simulink model "GCI_Ctrl_PLL_C2000"  (R2024a)
settings: Solver=FixedStepDiscrete  StartTime=0.0  StopTime=8  FixedStep=Sim.ContSampleTime  RelTol=1e-3  EnableMultiTasking=on
values from neighbouring files (symbols this model uses):
  ADPTV = 1.3912    [ModelDD.sldd]
  Ctrl = 0    [ModelDD.sldd]
  EnableMonitors = 0    [ModelDD.sldd]
  FrcPwr = 1    [ModelDD.sldd]
  IdSp = 0.0    [ModelDD.sldd]
  IqSp = 0.0    [ModelDD.sldd]
  ModReq = 1    [ModelDD.sldd]
  PorISel = 0    [ModelDD.sldd]
  PSp = 0.0    [ModelDD.sldd]
  QSp = 0.0    [ModelDD.sldd]
  Sim : value not decoded    [ModelDD.sldd]
  Test = 0    [ModelDD.sldd]
  Var = 650.0    [ModelDD.sldd]
undefined symbols (not defined in the file or in its folder): DiscIntNeverNeededParam, Down, GPTRIP1SEL, GPTRIP2SEL, magnitude, P, TZ1, TZ2, Up
libraries: simulink x38, c2837xDlib x22, c2802xlib x15, slpidlib x9, spsMeanLib x9, spsCurrentMeasurementLib x7, spsThreePhaseVIMeasurementLib x5, spsVoltageMeasurementLib x5, spsTHDLib x4, spsSeriesRLCBranchLib x4, svdutilitieslib x3, c280xlib x3
(part 10 of 11)

== system GCI_Ctrl_PLL_C2000/C2000_SW/CtrlLoop/CurrentController/CurrentControllerAdptv/Subsystem/dd_dqz1/LPF1 ==
  u : Inport
  Alpha : Gain  Gain=(2-w*Ts)/(2+w*Ts)
  Beta : Gain  Gain=(w*Ts)/(2+w*Ts)
  Delay1 : Delay  DelayLength=1  InitialCondition=y_0
  Delay2 : Delay  DelayLength=1
  Sum1 : Sum  Inputs=++|
  Sum2 : Sum  Inputs=|++
  y : Outport  VectorParamsAs1DForOutWhenUnconnected=off
  wires:
  u/1 -> Sum1/1, Delay2/1
  Delay1/1 -> Alpha/1  "y(n-1)"
  Alpha/1 -> Sum2/2
  Delay2/1 -> Sum1/2
  Sum1/1 -> Beta/1
  Beta/1 -> Sum2/1
  Sum2/1 -> Delay1/1, y/1

== system GCI_Ctrl_PLL_C2000/C2000_SW/CtrlLoop/CurrentController/CurrentControllerAdptv/Subsystem/dd_dqz1/Subsystem ==
  abc : Inport  PortDimensions=3
  Gain1 : Gain  Gain=single(2/3)  ParamDataTypeStr=single  SaturateOnIntegerOverflow=on  OutDataTypeStr=Inherit: Same as input
  Gain3 : Gain  Gain="single([ 1   -1/2   -1/2; 0   sqrt(3)/2   -sqrt(3)/2; 1/2  1/2  1/2 ] )"  Multiplication=Matrix(K*u) (u vector)  ParamDataTypeStr=single  SaturateOnIntegerOverflow=on  OutDataTypeStr=Inherit: Same as input
  al_be_0 : Outport  VectorParamsAs1DForOutWhenUnconnected=off
  wires:
  Gain1/1 -> al_be_0/1  "AlphaBetaZero"
  Gain3/1 -> Gain1/1
  abc/1 -> Gain3/1

== system GCI_Ctrl_PLL_C2000/C2000_SW/CtrlLoop/CurrentController/CurrentControllerAdptv/Subsystem/dd_dqz1/Subsystem1 ==
  note: [  al
      |     be  ]
  note: q = -al*sin(wt) + be*cos(wt)
  note: [  cos(wt)   sin(wt)
      |    -sin(wt)    cos(wt)   ]
  note: d = al*cos(wt) + be*sin(wt)
  note: [ d
      |    q ]
  note: *
  note: =
  alpha_beta : Inport
  wtNow : Inport  Port=2  PortDimensions=1
  Fcn : Fcn  Expr=u[1]*cos(u[3]) + u[2]*sin(u[3])
  Fcn1 : Fcn  Expr=-u[1]*sin(u[3]) + u[2]*cos(u[3])
  Mux : Mux  Inputs=3
  Mux1 : Mux  Inputs=[2 1]
  Mux2 : Mux  Inputs=[2 1]
  Selector : Selector  InputPortWidth=3  IndexOptions=Index vector (dialog)  Indices=[1 2]  OutputSizes=1
  Selector1 : Selector  InputPortWidth=3  IndexOptions=Index vector (dialog)  Indices=[3]  OutputSizes=1
  dq : Outport  InitialOutput=[0,0]  VectorParamsAs1DForOutWhenUnconnected=off
  wires:
  Selector1/1 -> Mux/3
  Selector/1 -> Mux1/1, Mux2/1
  Mux2/1 -> Fcn1/1
  Mux/1 -> dq/1
  wtNow/1 -> Mux1/2, Mux2/2
  Fcn/1 -> Mux/1
  Fcn1/1 -> Mux/2
  Mux1/1 -> Fcn/1
  alpha_beta/1 -> Selector1/1, Selector/1

== system GCI_Ctrl_PLL_C2000/C2000_SW/CtrlLoop/CurrentController/CurrentControllerAdptv/Subsystem/dd_dqz1/Subsystem2 ==
  note: =
  note: *
  note: [ d
      |    q ]
  note: d = al*cos(wt) + be*sin(wt)
  note: [  cos(wt)   sin(wt)
      |    -sin(wt)    cos(wt)   ]
  note: q = -al*sin(wt) + be*cos(wt)
  note: [  al
      |     be  ]
  alpha_beta : Inport
  wtNow : Inport  Port=2  PortDimensions=1
  Fcn : Fcn  Expr=u[1]*cos(u[3]) + u[2]*sin(u[3])
  Fcn1 : Fcn  Expr=-u[1]*sin(u[3]) + u[2]*cos(u[3])
  Mux : Mux  Inputs=3
  Mux1 : Mux  Inputs=[2 1]
  Mux2 : Mux  Inputs=[2 1]
  Selector : Selector  InputPortWidth=3  IndexOptions=Index vector (dialog)  Indices=[1 2]  OutputSizes=1
  Selector1 : Selector  InputPortWidth=3  IndexOptions=Index vector (dialog)  Indices=[3]  OutputSizes=1
  dq : Outport  InitialOutput=[0,0]  VectorParamsAs1DForOutWhenUnconnected=off
  wires:
  wtNow/1 -> Mux1/2, Mux2/2
  alpha_beta/1 -> Selector/1, Selector1/1
  Mux1/1 -> Fcn/1
  Fcn1/1 -> Mux/2
  Fcn/1 -> Mux/1
  Mux/1 -> dq/1
  Mux2/1 -> Fcn1/1
  Selector/1 -> Mux2/1, Mux1/1
  Selector1/1 -> Mux/3

== system GCI_Ctrl_PLL_C2000/C2000_SW/CtrlLoop/CurrentController/CurrentControllerAdptv/Subsystem/dd_dqz1/Subsystem3 ==
  Vdq_in : Inport
  Vdq_Inverse : Inport  Port=2
  Theta : Inport  Port=3
  Cos : Trigonometry  Operator=cos
  Cos1 : Trigonometry
  Demux1 : Demux  Outputs=2
  Demux2 : Demux  Outputs=2
  Gain : Gain  Gain=2  ParamDataTypeStr=single
  Ground : Ground
  Mux : Mux  Inputs=3
  Product{,1..3} (4 alike) : Product
  Selector : Selector  InputPortWidth=3  IndexOptions=Index vector (dialog)  Indices=[1 2]  OutputSizes=1
  Selector1 : Selector  InputPortWidth=3  IndexOptions=Index vector (dialog)  Indices=[1 2]  OutputSizes=1
  Sum : Sum  Inputs=|+-
  Sum1 : Sum  Inputs=|++
  Sum2 : Sum  Inputs=|+-
  Sum3 : Sum  Inputs=|+-
  Vdq_out : Outport  VectorParamsAs1DForOutWhenUnconnected=off
  wires:
  Theta/1 -> Gain/1
  Gain/1 -> Cos/1, Cos1/1
  Vdq_in/1 -> Selector/1
  Selector/1 -> Demux2/1
  Selector1/1 -> Demux1/1
  Vdq_Inverse/1 -> Selector1/1
  Demux2/1 -> [Vd_Pos]
  Demux2/2 -> [Vq_Pos]
  Demux1/1 -> [Vd_Neg]
  Demux1/2 -> [Vq_Neg]
  [Vd_Pos] -> Sum/1
  Cos1/1 -> [Sin]
  Cos/1 -> [Cos]
  Product/1 -> Sum/2
  [Vd_Neg] -> Product/1
  [Cos] -> Product/2
  [Sin] -> Product1/2
  [Vd_Neg] -> Product1/1
  Product1/1 -> Sum1/2
  [Vq_Pos] -> Sum1/1
  Sum/1 -> Sum2/1
  Sum2/1 -> Mux/1
  [Sin] -> Product2/2
  [Vq_Neg] -> Product2/1
  Product2/1 -> Sum2/2
  [Cos] -> Product3/2
  [Vq_Neg] -> Product3/1
  Sum1/1 -> Sum3/1
  Product3/1 -> Sum3/2
  Sum3/1 -> Mux/2
  Mux/1 -> Vdq_out/1
  Ground/1 -> Mux/3

== system GCI_Ctrl_PLL_C2000/C2000_SW/CtrlLoop/CurrentController/CurrentControllerAdptv/Subsystem/dd_dqz1/Subsystem4 ==
  Vdq_in : Inport
  Vdq_Inverse : Inport  Port=2
  Theta : Inport  Port=3
  Cos : Trigonometry  Operator=cos
  Cos1 : Trigonometry
  Demux1 : Demux  Outputs=2
  Demux2 : Demux  Outputs=2
  Gain : Gain  Gain=2  ParamDataTypeStr=single
  Ground : Ground
  Mux : Mux  Inputs=3
  Product{,1..3} (4 alike) : Product
  Selector : Selector  InputPortWidth=3  IndexOptions=Index vector (dialog)  Indices=[1 2]  OutputSizes=1
  Selector1 : Selector  InputPortWidth=3  IndexOptions=Index vector (dialog)  Indices=[1 2]  OutputSizes=1
  Sum : Sum  Inputs=|+-
  Sum1 : Sum  Inputs=|++
  Sum2 : Sum  Inputs=|+-
  Sum3 : Sum  Inputs=|+-
  Vdq_out : Outport  VectorParamsAs1DForOutWhenUnconnected=off
  wires:
  Ground/1 -> Mux/3
  Mux/1 -> Vdq_out/1
  Sum3/1 -> Mux/2
  Product3/1 -> Sum3/2
  Sum1/1 -> Sum3/1
  [Vq_Neg] -> Product3/1
  [Cos] -> Product3/2
  Product2/1 -> Sum2/2
  [Vq_Neg] -> Product2/1
  [Sin] -> Product2/2
  Sum2/1 -> Mux/1
  Sum/1 -> Sum2/1
  [Vq_Pos] -> Sum1/1
  Product1/1 -> Sum1/2
  [Vd_Neg] -> Product1/1
  [Sin] -> Product1/2
  [Cos] -> Product/2
  [Vd_Neg] -> Product/1
  Product/1 -> Sum/2
  Cos/1 -> [Cos]
  Cos1/1 -> [Sin]
  [Vd_Pos] -> Sum/1
  Demux1/2 -> [Vq_Neg]
  Demux1/1 -> [Vd_Neg]
  Demux2/2 -> [Vq_Pos]
  Demux2/1 -> [Vd_Pos]
  Vdq_Inverse/1 -> Selector1/1
  Selector1/1 -> Demux1/1
  Selector/1 -> Demux2/1
  Vdq_in/1 -> Selector/1
  Gain/1 -> Cos/1, Cos1/1
  Theta/1 -> Gain/1

== system GCI_Ctrl_PLL_C2000/C2000_SW/CtrlLoop/CurrentController/CurrentControllerAdptv/Subsystem/dd_dqz2/LPF ==
  u : Inport
  Alpha : Gain  Gain=(2-w*Ts)/(2+w*Ts)
  Beta : Gain  Gain=(w*Ts)/(2+w*Ts)
  Delay1 : Delay  DelayLength=1  InitialCondition=y_0
  Delay2 : Delay  DelayLength=1
  Sum1 : Sum  Inputs=++|
  Sum2 : Sum  Inputs=|++
  y : Outport  VectorParamsAs1DForOutWhenUnconnected=off
  wires:
  Sum2/1 -> y/1, Delay1/1
  Beta/1 -> Sum2/1
  Sum1/1 -> Beta/1
  Delay2/1 -> Sum1/2
  Alpha/1 -> Sum2/2
  Delay1/1 -> Alpha/1  "y(n-1)"
  u/1 -> Delay2/1, Sum1/1

== system GCI_Ctrl_PLL_C2000/C2000_SW/CtrlLoop/CurrentController/CurrentControllerAdptv/Subsystem/dd_dqz2/LPF1 ==
  u : Inport
  Alpha : Gain  Gain=(2-w*Ts)/(2+w*Ts)
  Beta : Gain  Gain=(w*Ts)/(2+w*Ts)
  Delay1 : Delay  DelayLength=1  InitialCondition=y_0
  Delay2 : Delay  DelayLength=1
  Sum1 : Sum  Inputs=++|
  Sum2 : Sum  Inputs=|++
  y : Outport  VectorParamsAs1DForOutWhenUnconnected=off
  wires:
  u/1 -> Sum1/1, Delay2/1
  Delay1/1 -> Alpha/1  "y(n-1)"
  Alpha/1 -> Sum2/2
  Delay2/1 -> Sum1/2
  Sum1/1 -> Beta/1
  Beta/1 -> Sum2/1
  Sum2/1 -> Delay1/1, y/1

== system GCI_Ctrl_PLL_C2000/C2000_SW/CtrlLoop/CurrentController/CurrentControllerAdptv/Subsystem/dd_dqz2/Subsystem ==
  abc : Inport  PortDimensions=3
  Gain1 : Gain  Gain=single(2/3)  ParamDataTypeStr=single  SaturateOnIntegerOverflow=on  OutDataTypeStr=Inherit: Same as input
  Gain3 : Gain  Gain="single([ 1   -1/2   -1/2; 0   sqrt(3)/2   -sqrt(3)/2; 1/2  1/2  1/2 ] )"  Multiplication=Matrix(K*u) (u vector)  ParamDataTypeStr=single  SaturateOnIntegerOverflow=on  OutDataTypeStr=Inherit: Same as input
  al_be_0 : Outport  VectorParamsAs1DForOutWhenUnconnected=off
  wires:
  abc/1 -> Gain3/1
  Gain3/1 -> Gain1/1
  Gain1/1 -> al_be_0/1  "AlphaBetaZero"

== system GCI_Ctrl_PLL_C2000/C2000_SW/CtrlLoop/CurrentController/CurrentControllerAdptv/Subsystem/dd_dqz2/Subsystem1 ==
  note: =
  note: *
  note: [ d
      |    q ]
  note: d = al*cos(wt) + be*sin(wt)
  note: [  cos(wt)   sin(wt)
      |    -sin(wt)    cos(wt)   ]
  note: q = -al*sin(wt) + be*cos(wt)
  note: [  al
      |     be  ]
  alpha_beta : Inport
  wtNow : Inport  Port=2  PortDimensions=1
  Fcn : Fcn  Expr=u[1]*cos(u[3]) + u[2]*sin(u[3])
  Fcn1 : Fcn  Expr=-u[1]*sin(u[3]) + u[2]*cos(u[3])
  Mux : Mux  Inputs=3
  Mux1 : Mux  Inputs=[2 1]
  Mux2 : Mux  Inputs=[2 1]
  Selector : Selector  InputPortWidth=3  IndexOptions=Index vector (dialog)  Indices=[1 2]  OutputSizes=1
  Selector1 : Selector  InputPortWidth=3  IndexOptions=Index vector (dialog)  Indices=[3]  OutputSizes=1
  dq : Outport  InitialOutput=[0,0]  VectorParamsAs1DForOutWhenUnconnected=off
  wires:
  alpha_beta/1 -> Selector/1, Selector1/1
  Mux1/1 -> Fcn/1
  Fcn1/1 -> Mux/2
  Fcn/1 -> Mux/1
  wtNow/1 -> Mux2/2, Mux1/2
  Mux/1 -> dq/1  "dq"
  Mux2/1 -> Fcn1/1
  Selector/1 -> Mux2/1, Mux1/1
  Selector1/1 -> Mux/3

== system GCI_Ctrl_PLL_C2000/C2000_SW/CtrlLoop/CurrentController/CurrentControllerAdptv/Subsystem/dd_dqz2/Subsystem2 ==
  note: [  al
      |     be  ]
  note: q = -al*sin(wt) + be*cos(wt)
  note: [  cos(wt)   sin(wt)
      |    -sin(wt)    cos(wt)   ]
  note: d = al*cos(wt) + be*sin(wt)
  note: [ d
      |    q ]
  note: *
  note: =
  alpha_beta : Inport
  wtNow : Inport  Port=2  PortDimensions=1
  Fcn : Fcn  Expr=u[1]*cos(u[3]) + u[2]*sin(u[3])
  Fcn1 : Fcn  Expr=-u[1]*sin(u[3]) + u[2]*cos(u[3])
  Mux : Mux  Inputs=3
  Mux1 : Mux  Inputs=[2 1]
  Mux2 : Mux  Inputs=[2 1]
  Selector : Selector  InputPortWidth=3  IndexOptions=Index vector (dialog)  Indices=[1 2]  OutputSizes=1
  Selector1 : Selector  InputPortWidth=3  IndexOptions=Index vector (dialog)  Indices=[3]  OutputSizes=1
  dq : Outport  InitialOutput=[0,0]  VectorParamsAs1DForOutWhenUnconnected=off
  wires:
  Selector1/1 -> Mux/3
  Selector/1 -> Mux1/1, Mux2/1
  Mux2/1 -> Fcn1/1
  Mux/1 -> dq/1  "dq"
  wtNow/1 -> Mux1/2, Mux2/2
  Fcn/1 -> Mux/1
  Fcn1/1 -> Mux/2
  Mux1/1 -> Fcn/1
  alpha_beta/1 -> Selector1/1, Selector/1

== system GCI_Ctrl_PLL_C2000/C2000_SW/CtrlLoop/CurrentController/CurrentControllerAdptv/Subsystem/dd_dqz2/Subsystem3 ==
  Vdq_in : Inport
  Vdq_Inverse : Inport  Port=2
  Theta : Inport  Port=3
  Cos : Trigonometry  Operator=cos
  Demux1 : Demux  Outputs=2
  Demux2 : Demux  Outputs=2
  Gain : Gain  Gain=2  ParamDataTypeStr=single
  Ground : Ground
  Mux : Mux  Inputs=3
  Product{,1..3} (4 alike) : Product
  Selector : Selector  InputPortWidth=3  IndexOptions=Index vector (dialog)  Indices=[1 2]  OutputSizes=1
  Selector1 : Selector  InputPortWidth=3  IndexOptions=Index vector (dialog)  Indices=[1 2]  OutputSizes=1
  Sin : Trigonometry
  Sum : Sum  Inputs=|+-
  Sum1 : Sum  Inputs=|++
  Sum2 : Sum  Inputs=|+-
  Sum3 : Sum  Inputs=|+-
  Vdq_out : Outport  VectorParamsAs1DForOutWhenUnconnected=off
  wires:
  Ground/1 -> Mux/3
  Mux/1 -> Vdq_out/1
  Sum3/1 -> Mux/2
  Product3/1 -> Sum3/2
  Sum1/1 -> Sum3/1
  [Vq_Neg] -> Product3/1
  [Cos] -> Product3/2
  Product2/1 -> Sum2/2
  [Vq_Neg] -> Product2/1
  [Sin] -> Product2/2
  Sum2/1 -> Mux/1
  Sum/1 -> Sum2/1
  [Vq_Pos] -> Sum1/1
  Product1/1 -> Sum1/2
  [Vd_Neg] -> Product1/1
  [Sin] -> Product1/2
  [Cos] -> Product/2
  [Vd_Neg] -> Product/1
  Product/1 -> Sum/2
  Cos/1 -> [Cos]
  Sin/1 -> [Sin]
  [Vd_Pos] -> Sum/1
  Demux1/2 -> [Vq_Neg]
  Demux1/1 -> [Vd_Neg]
  Demux2/2 -> [Vq_Pos]
  Demux2/1 -> [Vd_Pos]
  Vdq_Inverse/1 -> Selector1/1
  Selector1/1 -> Demux1/1
  Selector/1 -> Demux2/1
  Vdq_in/1 -> Selector/1
  Gain/1 -> Sin/1, Cos/1
  Theta/1 -> Gain/1

== system GCI_Ctrl_PLL_C2000/C2000_SW/CtrlLoop/CurrentController/CurrentControllerAdptv/Subsystem/dd_dqz2/Subsystem4 ==
  Vdq_in : Inport
  Vdq_Inverse : Inport  Port=2
  Theta : Inport  Port=3
  Cos : Trigonometry  Operator=cos
  Demux1 : Demux  Outputs=2
  Demux2 : Demux  Outputs=2
  Gain : Gain  Gain=2  ParamDataTypeStr=single
  Ground : Ground
  Mux : Mux  Inputs=3
  Product{,1..3} (4 alike) : Product
  Selector : Selector  InputPortWidth=3  IndexOptions=Index vector (dialog)  Indices=[1 2]  OutputSizes=1
  Selector1 : Selector  InputPortWidth=3  IndexOptions=Index vector (dialog)  Indices=[1 2]  OutputSizes=1
  Sin : Trigonometry
  Sum : Sum  Inputs=|+-
  Sum1 : Sum  Inputs=|++
  Sum2 : Sum  Inputs=|+-
  Sum3 : Sum  Inputs=|+-
  Vdq_out : Outport  VectorParamsAs1DForOutWhenUnconnected=off
  wires:
  Theta/1 -> Gain/1
  Gain/1 -> Cos/1, Sin/1
  Vdq_in/1 -> Selector/1
  Selector/1 -> Demux2/1
  Selector1/1 -> Demux1/1
  Vdq_Inverse/1 -> Selector1/1
  Demux2/1 -> [Vd_Pos]
  Demux2/2 -> [Vq_Pos]
  Demux1/1 -> [Vd_Neg]
  Demux1/2 -> [Vq_Neg]
  [Vd_Pos] -> Sum/1
  Sin/1 -> [Sin]
  Cos/1 -> [Cos]
  Product/1 -> Sum/2
  [Vd_Neg] -> Product/1
  [Cos] -> Product/2
  [Sin] -> Product1/2
  [Vd_Neg] -> Product1/1
  Product1/1 -> Sum1/2
  [Vq_Pos] -> Sum1/1
  Sum/1 -> Sum2/1
  Sum2/1 -> Mux/1
  [Sin] -> Product2/2
  [Vq_Neg] -> Product2/1
  Product2/1 -> Sum2/2
  [Cos] -> Product3/2
  [Vq_Neg] -> Product3/1
  Sum1/1 -> Sum3/1
  Product3/1 -> Sum3/2
  Sum3/1 -> Mux/2
  Mux/1 -> Vdq_out/1
  Ground/1 -> Mux/3

== system GCI_Ctrl_PLL_C2000/C2000_SW/CtrlLoop/CurrentController/CurrentControllerAdptv2/MESO/CFDL/Mag ==
  In1 : Inport
  Reshape : Reshape
  Sqrt : Sqrt
  Square : Math  Operator=square
  Sum of Elements : Sum  Inputs=+
  Out1 : Outport
  wires:
  In1/1 -> Square/1
  Square/1 -> Sum of Elements/1
  Sum of Elements/1 -> Sqrt/1
  Sqrt/1 -> Reshape/1
  Reshape/1 -> Out1/1

== system GCI_Ctrl_PLL_C2000/C2000_SW/CtrlLoop/CurrentController/CurrentControllerAdptv2/MESO/Deso/Mag ==
  e_k : Inport
  Sqrt : Sqrt
  Square : Math  Operator=square
  Sum of Elements : Sum  Inputs=+
  Out1 : Outport
  wires:
  e_k/1 -> Square/1
  Square/1 -> Sum of Elements/1
  Sum of Elements/1 -> Sqrt/1
  Sqrt/1 -> Out1/1

== system GCI_Ctrl_PLL_C2000/C2000_SW/CtrlLoop/CurrentController/CurrentControllerAdptv2/MESO/Deso/Mag1 ==
  e_k : Inport
  Reshape : Reshape
  Sqrt : Sqrt
  Square : Math  Operator=square
  Sum of Elements : Sum  Inputs=+
  Out1 : Outport
  wires:
  Reshape/1 -> Out1/1
  Sqrt/1 -> Reshape/1
  Sum of Elements/1 -> Sqrt/1
  Square/1 -> Sum of Elements/1
  e_k/1 -> Square/1

== system GCI_Ctrl_PLL_C2000/C2000_SW/CtrlLoop/CurrentController/CurrentControllerAdptv2/Subsystem/abc_dqz/Subsystem ==
  abc : Inport  PortDimensions=3
  Gain1 : Gain  Gain=single(2/3)  ParamDataTypeStr=single  SaturateOnIntegerOverflow=on  OutDataTypeStr=Inherit: Same as input
  Gain3 : Gain  Gain="single([ 1   -1/2   -1/2; 0   sqrt(3)/2   -sqrt(3)/2; 1/2  1/2  1/2 ] )"  Multiplication=Matrix(K*u) (u vector)  ParamDataTypeStr=single  SaturateOnIntegerOverflow=on  OutDataTypeStr=Inherit: Same as input
  al_be_0 : Outport  VectorParamsAs1DForOutWhenUnconnected=off
  wires:
  abc/1 -> Gain3/1
  Gain3/1 -> Gain1/1
  Gain1/1 -> al_be_0/1

== system GCI_Ctrl_PLL_C2000/C2000_SW/CtrlLoop/CurrentController/CurrentControllerAdptv2/Subsystem/abc_dqz/Subsystem2 ==
  note: [  al
      |     be  ]
  note: q = -al*sin(wt) + be*cos(wt)
  note: [  cos(wt)   sin(wt)
      |    -sin(wt)    cos(wt)   ]
  note: d = al*cos(wt) + be*sin(wt)
  note: [ d
      |    q ]
  note: *
  note: =
  alpha_beta : Inport
  Ang : Inport  Port=2  PortDimensions=1
  Fcn : Fcn  Expr=u[1]*cos(u[3]) + u[2]*sin(u[3])
  Fcn1 : Fcn  Expr=-u[1]*sin(u[3]) + u[2]*cos(u[3])
  Mux : Mux  Inputs=3
  Mux1 : Mux  Inputs=[2 1]
  Mux2 : Mux  Inputs=[2 1]
  Selector : Selector  InputPortWidth=3  IndexOptions=Index vector (dialog)  Indices=[1 2]  OutputSizes=1
  Selector1 : Selector  InputPortWidth=3  IndexOptions=Index vector (dialog)  Indices=[3]  OutputSizes=1
  dq : Outport  InitialOutput=[0,0]  VectorParamsAs1DForOutWhenUnconnected=off
  wires:
  Selector1/1 -> Mux/3
  Selector/1 -> Mux1/1, Mux2/1
  Mux2/1 -> Fcn1/1
  Mux/1 -> dq/1
  Ang/1 -> Mux1/2, Mux2/2
  Fcn/1 -> Mux/1
  Fcn1/1 -> Mux/2
  Mux1/1 -> Fcn/1
  alpha_beta/1 -> Selector1/1, Selector/1

== system GCI_Ctrl_PLL_C2000/C2000_SW/CtrlLoop/CurrentController/CurrentControllerAdptv2/Subsystem/abc_dqz1/Subsystem ==
  abc : Inport  PortDimensions=3
  Gain1 : Gain  Gain=single(2/3)  ParamDataTypeStr=single  SaturateOnIntegerOverflow=on  OutDataTypeStr=Inherit: Same as input
  Gain3 : Gain  Gain="single([ 1   -1/2   -1/2; 0   sqrt(3)/2   -sqrt(3)/2; 1/2  1/2  1/2 ] )"  Multiplication=Matrix(K*u) (u vector)  ParamDataTypeStr=single  SaturateOnIntegerOverflow=on  OutDataTypeStr=Inherit: Same as input
  al_be_0 : Outport  VectorParamsAs1DForOutWhenUnconnected=off
  wires:
  Gain1/1 -> al_be_0/1
  Gain3/1 -> Gain1/1
  abc/1 -> Gain3/1

== system GCI_Ctrl_PLL_C2000/C2000_SW/CtrlLoop/CurrentController/CurrentControllerAdptv2/Subsystem/abc_dqz1/Subsystem2 ==
  note: =
  note: *
  note: [ d
      |    q ]
  note: d = al*cos(wt) + be*sin(wt)
  note: [  cos(wt)   sin(wt)
      |    -sin(wt)    cos(wt)   ]
  note: q = -al*sin(wt) + be*cos(wt)
  note: [  al
      |     be  ]
  alpha_beta : Inport
  Ang : Inport  Port=2  PortDimensions=1
  Fcn : Fcn  Expr=u[1]*cos(u[3]) + u[2]*sin(u[3])
  Fcn1 : Fcn  Expr=-u[1]*sin(u[3]) + u[2]*cos(u[3])
  Mux : Mux  Inputs=3
  Mux1 : Mux  Inputs=[2 1]
  Mux2 : Mux  Inputs=[2 1]
  Selector : Selector  InputPortWidth=3  IndexOptions=Index vector (dialog)  Indices=[1 2]  OutputSizes=1
  Selector1 : Selector  InputPortWidth=3  IndexOptions=Index vector (dialog)  Indices=[3]  OutputSizes=1
  dq : Outport  InitialOutput=[0,0]  VectorParamsAs1DForOutWhenUnconnected=off
  wires:
  alpha_beta/1 -> Selector/1, Selector1/1
  Mux1/1 -> Fcn/1
  Fcn1/1 -> Mux/2
  Fcn/1 -> Mux/1
  Ang/1 -> Mux2/2, Mux1/2
  Mux/1 -> dq/1
  Mux2/1 -> Fcn1/1
  Selector/1 -> Mux2/1, Mux1/1
  Selector1/1 -> Mux/3

== system GCI_Ctrl_PLL_C2000/C2000_SW/CtrlLoop/CurrentController/CurrentControllerAdptv2/Subsystem/dd_dqz1/LPF ==
  u : Inport
  Alpha : Gain  Gain=(2-w*Ts)/(2+w*Ts)
  Beta : Gain  Gain=(w*Ts)/(2+w*Ts)
  Delay1 : Delay  DelayLength=1  InitialCondition=y_0
  Delay2 : Delay  DelayLength=1
  Sum1 : Sum  Inputs=++|
  Sum2 : Sum  Inputs=|++
  y : Outport  VectorParamsAs1DForOutWhenUnconnected=off
  wires:
  u/1 -> Sum1/1, Delay2/1
  Delay1/1 -> Alpha/1  "y(n-1)"
  Alpha/1 -> Sum2/2
  Delay2/1 -> Sum1/2
  Sum1/1 -> Beta/1
  Beta/1 -> Sum2/1
  Sum2/1 -> Delay1/1, y/1

== system GCI_Ctrl_PLL_C2000/C2000_SW/CtrlLoop/CurrentController/CurrentControllerAdptv2/Subsystem/dd_dqz1/LPF1 ==
  u : Inport
  Alpha : Gain  Gain=(2-w*Ts)/(2+w*Ts)
  Beta : Gain  Gain=(w*Ts)/(2+w*Ts)
  Delay1 : Delay  DelayLength=1  InitialCondition=y_0
  Delay2 : Delay  DelayLength=1
  Sum1 : Sum  Inputs=++|
  Sum2 : Sum  Inputs=|++
  y : Outport  VectorParamsAs1DForOutWhenUnconnected=off
  wires:
  Sum2/1 -> y/1, Delay1/1
  Beta/1 -> Sum2/1
  Sum1/1 -> Beta/1
  Delay2/1 -> Sum1/2
  Alpha/1 -> Sum2/2
  Delay1/1 -> Alpha/1  "y(n-1)"
  u/1 -> Delay2/1, Sum1/1

== system GCI_Ctrl_PLL_C2000/C2000_SW/CtrlLoop/CurrentController/CurrentControllerAdptv2/Subsystem/dd_dqz1/Subsystem ==
  abc : Inport  PortDimensions=3
  Gain1 : Gain  Gain=single(2/3)  ParamDataTypeStr=single  SaturateOnIntegerOverflow=on  OutDataTypeStr=Inherit: Same as input
  Gain3 : Gain  Gain="single([ 1   -1/2   -1/2; 0   sqrt(3)/2   -sqrt(3)/2; 1/2  1/2  1/2 ] )"  Multiplication=Matrix(K*u) (u vector)  ParamDataTypeStr=single  SaturateOnIntegerOverflow=on  OutDataTypeStr=Inherit: Same as input
  al_be_0 : Outport  VectorParamsAs1DForOutWhenUnconnected=off
  wires:
  abc/1 -> Gain3/1
  Gain3/1 -> Gain1/1
  Gain1/1 -> al_be_0/1  "AlphaBetaZero"

== system GCI_Ctrl_PLL_C2000/C2000_SW/CtrlLoop/CurrentController/CurrentControllerAdptv2/Subsystem/dd_dqz1/Subsystem1 ==
  note: =
  note: *
  note: [ d
      |    q ]
  note: d = al*cos(wt) + be*sin(wt)
  note: [  cos(wt)   sin(wt)
      |    -sin(wt)    cos(wt)   ]
  note: q = -al*sin(wt) + be*cos(wt)
  note: [  al
      |     be  ]
  alpha_beta : Inport
  wtNow : Inport  Port=2  PortDimensions=1
  Fcn : Fcn  Expr=u[1]*cos(u[3]) + u[2]*sin(u[3])
  Fcn1 : Fcn  Expr=-u[1]*sin(u[3]) + u[2]*cos(u[3])
  Mux : Mux  Inputs=3
  Mux1 : Mux  Inputs=[2 1]
  Mux2 : Mux  Inputs=[2 1]
  Selector : Selector  InputPortWidth=3  IndexOptions=Index vector (dialog)  Indices=[1 2]  OutputSizes=1
  Selector1 : Selector  InputPortWidth=3  IndexOptions=Index vector (dialog)  Indices=[3]  OutputSizes=1
  dq : Outport  InitialOutput=[0,0]  VectorParamsAs1DForOutWhenUnconnected=off
  wires:
  alpha_beta/1 -> Selector/1, Selector1/1
  Mux1/1 -> Fcn/1
  Fcn1/1 -> Mux/2
  Fcn/1 -> Mux/1
  wtNow/1 -> Mux2/2, Mux1/2
  Mux/1 -> dq/1
  Mux2/1 -> Fcn1/1
  Selector/1 -> Mux2/1, Mux1/1
  Selector1/1 -> Mux/3

== system GCI_Ctrl_PLL_C2000/C2000_SW/CtrlLoop/CurrentController/CurrentControllerAdptv2/Subsystem/dd_dqz1/Subsystem2 ==
  note: [  al
      |     be  ]
  note: q = -al*sin(wt) + be*cos(wt)
  note: [  cos(wt)   sin(wt)
      |    -sin(wt)    cos(wt)   ]
  note: d = al*cos(wt) + be*sin(wt)
  note: [ d
      |    q ]
  note: *
  note: =
  alpha_beta : Inport
  wtNow : Inport  Port=2  PortDimensions=1
  Fcn : Fcn  Expr=u[1]*cos(u[3]) + u[2]*sin(u[3])
  Fcn1 : Fcn  Expr=-u[1]*sin(u[3]) + u[2]*cos(u[3])
  Mux : Mux  Inputs=3
  Mux1 : Mux  Inputs=[2 1]
  Mux2 : Mux  Inputs=[2 1]
  Selector : Selector  InputPortWidth=3  IndexOptions=Index vector (dialog)  Indices=[1 2]  OutputSizes=1
  Selector1 : Selector  InputPortWidth=3  IndexOptions=Index vector (dialog)  Indices=[3]  OutputSizes=1
  dq : Outport  InitialOutput=[0,0]  VectorParamsAs1DForOutWhenUnconnected=off
  wires:
  Selector1/1 -> Mux/3
  Selector/1 -> Mux1/1, Mux2/1
  Mux2/1 -> Fcn1/1
  Mux/1 -> dq/1
  Fcn/1 -> Mux/1
  Fcn1/1 -> Mux/2
  Mux1/1 -> Fcn/1
  alpha_beta/1 -> Selector1/1, Selector/1
  wtNow/1 -> Mux2/2, Mux1/2

== system GCI_Ctrl_PLL_C2000/C2000_SW/CtrlLoop/CurrentController/CurrentControllerAdptv2/Subsystem/dd_dqz1/Subsystem3 ==
  Vdq_in : Inport
  Vdq_Inverse : Inport  Port=2
  Theta : Inport  Port=3
  Cos : Trigonometry  Operator=cos
  Cos1 : Trigonometry
  Demux1 : Demux  Outputs=2
  Demux2 : Demux  Outputs=2
  Gain : Gain  Gain=2  ParamDataTypeStr=single
  Ground : Ground
  Mux : Mux  Inputs=3
  Product{,1..3} (4 alike) : Product
  Selector : Selector  InputPortWidth=3  IndexOptions=Index vector (dialog)  Indices=[1 2]  OutputSizes=1
  Selector1 : Selector  InputPortWidth=3  IndexOptions=Index vector (dialog)  Indices=[1 2]  OutputSizes=1
  Sum : Sum  Inputs=|+-
  Sum1 : Sum  Inputs=|++
  Sum2 : Sum  Inputs=|+-
  Sum3 : Sum  Inputs=|+-
  Vdq_out : Outport  VectorParamsAs1DForOutWhenUnconnected=off
  wires:
  Ground/1 -> Mux/3
  Mux/1 -> Vdq_out/1
  Sum3/1 -> Mux/2
  Product3/1 -> Sum3/2
  Sum1/1 -> Sum3/1
  [Vq_Neg] -> Product3/1
  [Cos] -> Product3/2
  Product2/1 -> Sum2/2
  [Vq_Neg] -> Product2/1
  [Sin] -> Product2/2
  Sum2/1 -> Mux/1
  Sum/1 -> Sum2/1
  [Vq_Pos] -> Sum1/1
  Product1/1 -> Sum1/2
  [Vd_Neg] -> Product1/1
  [Sin] -> Product1/2
  [Cos] -> Product/2
  [Vd_Neg] -> Product/1
  Product/1 -> Sum/2
  Cos/1 -> [Cos]
  Cos1/1 -> [Sin]
  [Vd_Pos] -> Sum/1
  Demux1/2 -> [Vq_Neg]
  Demux1/1 -> [Vd_Neg]
  Demux2/2 -> [Vq_Pos]
  Demux2/1 -> [Vd_Pos]
  Vdq_Inverse/1 -> Selector1/1
  Selector1/1 -> Demux1/1
  Selector/1 -> Demux2/1
  Vdq_in/1 -> Selector/1
  Gain/1 -> Cos1/1, Cos/1
  Theta/1 -> Gain/1

== system GCI_Ctrl_PLL_C2000/C2000_SW/CtrlLoop/CurrentController/CurrentControllerAdptv2/Subsystem/dd_dqz1/Subsystem4 ==
  Vdq_in : Inport
  Vdq_Inverse : Inport  Port=2
  Theta : Inport  Port=3
  Cos : Trigonometry  Operator=cos
  Cos1 : Trigonometry
  Demux1 : Demux  Outputs=2
  Demux2 : Demux  Outputs=2
  Gain : Gain  Gain=2  ParamDataTypeStr=single
  Ground : Ground
  Mux : Mux  Inputs=3
  Product{,1..3} (4 alike) : Product
  Selector : Selector  InputPortWidth=3  IndexOptions=Index vector (dialog)  Indices=[1 2]  OutputSizes=1
  Selector1 : Selector  InputPortWidth=3  IndexOptions=Index vector (dialog)  Indices=[1 2]  OutputSizes=1
  Sum : Sum  Inputs=|+-
  Sum1 : Sum  Inputs=|++
  Sum2 : Sum  Inputs=|+-
  Sum3 : Sum  Inputs=|+-
  Vdq_out : Outport  VectorParamsAs1DForOutWhenUnconnected=off
  wires:
  Theta/1 -> Gain/1
  Gain/1 -> Cos1/1, Cos/1
  Vdq_in/1 -> Selector/1
  Selector/1 -> Demux2/1
  Selector1/1 -> Demux1/1
  Vdq_Inverse/1 -> Selector1/1
  Demux2/1 -> [Vd_Pos]
  Demux2/2 -> [Vq_Pos]
  Demux1/1 -> [Vd_Neg]
  Demux1/2 -> [Vq_Neg]
  [Vd_Pos] -> Sum/1
  Cos1/1 -> [Sin]
  Cos/1 -> [Cos]
  Product/1 -> Sum/2
  [Vd_Neg] -> Product/1
  [Cos] -> Product/2
  [Sin] -> Product1/2
  [Vd_Neg] -> Product1/1
  Product1/1 -> Sum1/2
  [Vq_Pos] -> Sum1/1
  Sum/1 -> Sum2/1
  Sum2/1 -> Mux/1
  [Sin] -> Product2/2
  [Vq_Neg] -> Product2/1
  Product2/1 -> Sum2/2
  [Cos] -> Product3/2
  [Vq_Neg] -> Product3/1
  Sum1/1 -> Sum3/1
  Product3/1 -> Sum3/2
  Sum3/1 -> Mux/2
  Mux/1 -> Vdq_out/1
  Ground/1 -> Mux/3

== system GCI_Ctrl_PLL_C2000/C2000_SW/CtrlLoop/CurrentController/CurrentControllerAdptv2/Subsystem/dd_dqz2/LPF ==
  u : Inport
  Alpha : Gain  Gain=(2-w*Ts)/(2+w*Ts)
  Beta : Gain  Gain=(w*Ts)/(2+w*Ts)
  Delay1 : Delay  DelayLength=1  InitialCondition=y_0
  Delay2 : Delay  DelayLength=1
  Sum1 : Sum  Inputs=++|
  Sum2 : Sum  Inputs=|++
  y : Outport  VectorParamsAs1DForOutWhenUnconnected=off
  wires:
  u/1 -> Sum1/1, Delay2/1
  Delay1/1 -> Alpha/1  "y(n-1)"
  Alpha/1 -> Sum2/2
  Delay2/1 -> Sum1/2
  Sum1/1 -> Beta/1
  Beta/1 -> Sum2/1
  Sum2/1 -> Delay1/1, y/1

== system GCI_Ctrl_PLL_C2000/C2000_SW/CtrlLoop/CurrentController/CurrentControllerAdptv2/Subsystem/dd_dqz2/LPF1 ==
  u : Inport
  Alpha : Gain  Gain=(2-w*Ts)/(2+w*Ts)
  Beta : Gain  Gain=(w*Ts)/(2+w*Ts)
  Delay1 : Delay  DelayLength=1  InitialCondition=y_0
  Delay2 : Delay  DelayLength=1
  Sum1 : Sum  Inputs=++|
  Sum2 : Sum  Inputs=|++
  y : Outport  VectorParamsAs1DForOutWhenUnconnected=off
  wires:
  Sum2/1 -> y/1, Delay1/1
  Beta/1 -> Sum2/1
  Sum1/1 -> Beta/1
  Delay2/1 -> Sum1/2
  Alpha/1 -> Sum2/2
  Delay1/1 -> Alpha/1  "y(n-1)"
  u/1 -> Delay2/1, Sum1/1

== system GCI_Ctrl_PLL_C2000/C2000_SW/CtrlLoop/CurrentController/CurrentControllerAdptv2/Subsystem/dd_dqz2/Subsystem ==
  abc : Inport  PortDimensions=3
  Gain1 : Gain  Gain=single(2/3)  ParamDataTypeStr=single  SaturateOnIntegerOverflow=on  OutDataTypeStr=Inherit: Same as input
  Gain3 : Gain  Gain="single([ 1   -1/2   -1/2; 0   sqrt(3)/2   -sqrt(3)/2; 1/2  1/2  1/2 ] )"  Multiplication=Matrix(K*u) (u vector)  ParamDataTypeStr=single  SaturateOnIntegerOverflow=on  OutDataTypeStr=Inherit: Same as input
  al_be_0 : Outport  VectorParamsAs1DForOutWhenUnconnected=off
  wires:
  Gain1/1 -> al_be_0/1  "AlphaBetaZero"
  Gain3/1 -> Gain1/1
  abc/1 -> Gain3/1

== system GCI_Ctrl_PLL_C2000/C2000_SW/CtrlLoop/CurrentController/CurrentControllerAdptv2/Subsystem/dd_dqz2/Subsystem1 ==
  note: [  al
      |     be  ]
  note: q = -al*sin(wt) + be*cos(wt)
  note: [  cos(wt)   sin(wt)
      |    -sin(wt)    cos(wt)   ]
  note: d = al*cos(wt) + be*sin(wt)
  note: [ d
      |    q ]
  note: *
  note: =
  alpha_beta : Inport
  wtNow : Inport  Port=2  PortDimensions=1
  Fcn : Fcn  Expr=u[1]*cos(u[3]) + u[2]*sin(u[3])
  Fcn1 : Fcn  Expr=-u[1]*sin(u[3]) + u[2]*cos(u[3])
  Mux : Mux  Inputs=3
  Mux1 : Mux  Inputs=[2 1]
  Mux2 : Mux  Inputs=[2 1]
  Selector : Selector  InputPortWidth=3  IndexOptions=Index vector (dialog)  Indices=[1 2]  OutputSizes=1
  Selector1 : Selector  InputPortWidth=3  IndexOptions=Index vector (dialog)  Indices=[3]  OutputSizes=1
  dq : Outport  InitialOutput=[0,0]  VectorParamsAs1DForOutWhenUnconnected=off
  wires:
  Selector1/1 -> Mux/3
  Selector/1 -> Mux1/1, Mux2/1
  Mux2/1 -> Fcn1/1
  Mux/1 -> dq/1  "dq"
  wtNow/1 -> Mux1/2, Mux2/2
  Fcn/1 -> Mux/1
  Fcn1/1 -> Mux/2
  Mux1/1 -> Fcn/1
  alpha_beta/1 -> Selector1/1, Selector/1

== system GCI_Ctrl_PLL_C2000/C2000_SW/CtrlLoop/CurrentController/CurrentControllerAdptv2/Subsystem/dd_dqz2/Subsystem2 ==
  note: =
  note: *
  note: [ d
      |    q ]
  note: d = al*cos(wt) + be*sin(wt)
  note: [  cos(wt)   sin(wt)
      |    -sin(wt)    cos(wt)   ]
  note: q = -al*sin(wt) + be*cos(wt)
  note: [  al
      |     be  ]
  alpha_beta : Inport
  wtNow : Inport  Port=2  PortDimensions=1
  Fcn : Fcn  Expr=u[1]*cos(u[3]) + u[2]*sin(u[3])
  Fcn1 : Fcn  Expr=-u[1]*sin(u[3]) + u[2]*cos(u[3])
  Mux : Mux  Inputs=3
  Mux1 : Mux  Inputs=[2 1]
  Mux2 : Mux  Inputs=[2 1]
  Selector : Selector  InputPortWidth=3  IndexOptions=Index vector (dialog)  Indices=[1 2]  OutputSizes=1
  Selector1 : Selector  InputPortWidth=3  IndexOptions=Index vector (dialog)  Indices=[3]  OutputSizes=1
  dq : Outport  InitialOutput=[0,0]  VectorParamsAs1DForOutWhenUnconnected=off
  wires:
  alpha_beta/1 -> Selector/1, Selector1/1
  Mux1/1 -> Fcn/1
  Fcn1/1 -> Mux/2
  Fcn/1 -> Mux/1
  wtNow/1 -> Mux2/2, Mux1/2
  Mux/1 -> dq/1  "dq"
  Mux2/1 -> Fcn1/1
  Selector/1 -> Mux2/1, Mux1/1
  Selector1/1 -> Mux/3

== system GCI_Ctrl_PLL_C2000/C2000_SW/CtrlLoop/CurrentController/CurrentControllerAdptv2/Subsystem/dd_dqz2/Subsystem3 ==
  Vdq_in : Inport
  Vdq_Inverse : Inport  Port=2
  Theta : Inport  Port=3
  Cos : Trigonometry  Operator=cos
  Demux1 : Demux  Outputs=2
  Demux2 : Demux  Outputs=2
  Gain : Gain  Gain=2  ParamDataTypeStr=single
  Ground : Ground
  Mux : Mux  Inputs=3
  Product{,1..3} (4 alike) : Product
  Selector : Selector  InputPortWidth=3  IndexOptions=Index vector (dialog)  Indices=[1 2]  OutputSizes=1
  Selector1 : Selector  InputPortWidth=3  IndexOptions=Index vector (dialog)  Indices=[1 2]  OutputSizes=1
  Sin : Trigonometry
  Sum : Sum  Inputs=|+-
  Sum1 : Sum  Inputs=|++
  Sum2 : Sum  Inputs=|+-
  Sum3 : Sum  Inputs=|+-
  Vdq_out : Outport  VectorParamsAs1DForOutWhenUnconnected=off
  wires:
  Theta/1 -> Gain/1
  Gain/1 -> Cos/1, Sin/1
  Vdq_in/1 -> Selector/1
  Selector/1 -> Demux2/1
  Selector1/1 -> Demux1/1
  Vdq_Inverse/1 -> Selector1/1
  Demux2/1 -> [Vd_Pos]
  Demux2/2 -> [Vq_Pos]
  Demux1/1 -> [Vd_Neg]
  Demux1/2 -> [Vq_Neg]
  [Vd_Pos] -> Sum/1
  Sin/1 -> [Sin]
  Cos/1 -> [Cos]
  Product/1 -> Sum/2
  [Vd_Neg] -> Product/1
  [Cos] -> Product/2
  [Sin] -> Product1/2
  [Vd_Neg] -> Product1/1
  Product1/1 -> Sum1/2
  [Vq_Pos] -> Sum1/1
  Sum/1 -> Sum2/1
  Sum2/1 -> Mux/1
  [Sin] -> Product2/2
  [Vq_Neg] -> Product2/1
  Product2/1 -> Sum2/2
  [Cos] -> Product3/2
  [Vq_Neg] -> Product3/1
  Sum1/1 -> Sum3/1
  Product3/1 -> Sum3/2
  Sum3/1 -> Mux/2
  Mux/1 -> Vdq_out/1
  Ground/1 -> Mux/3

== system GCI_Ctrl_PLL_C2000/C2000_SW/CtrlLoop/CurrentController/CurrentControllerAdptv2/Subsystem/dd_dqz2/Subsystem4 ==
  Vdq_in : Inport
  Vdq_Inverse : Inport  Port=2
  Theta : Inport  Port=3
  Cos : Trigonometry  Operator=cos
  Demux1 : Demux  Outputs=2
  Demux2 : Demux  Outputs=2
  Gain : Gain  Gain=2  ParamDataTypeStr=single
  Ground : Ground
  Mux : Mux  Inputs=3
  Product{,1..3} (4 alike) : Product
  Selector : Selector  InputPortWidth=3  IndexOptions=Index vector (dialog)  Indices=[1 2]  OutputSizes=1
  Selector1 : Selector  InputPortWidth=3  IndexOptions=Index vector (dialog)  Indices=[1 2]  OutputSizes=1
  Sin : Trigonometry
  Sum : Sum  Inputs=|+-
  Sum1 : Sum  Inputs=|++
  Sum2 : Sum  Inputs=|+-
  Sum3 : Sum  Inputs=|+-
  Vdq_out : Outport  VectorParamsAs1DForOutWhenUnconnected=off
  wires:
  Ground/1 -> Mux/3
  Mux/1 -> Vdq_out/1
  Sum3/1 -> Mux/2
  Product3/1 -> Sum3/2
  Sum1/1 -> Sum3/1
  [Vq_Neg] -> Product3/1
  [Cos] -> Product3/2
  Product2/1 -> Sum2/2
  [Vq_Neg] -> Product2/1
  [Sin] -> Product2/2
  Sum2/1 -> Mux/1
  Sum/1 -> Sum2/1
  [Vq_Pos] -> Sum1/1
  Product1/1 -> Sum1/2
  [Vd_Neg] -> Product1/1
  [Sin] -> Product1/2
  [Cos] -> Product/2
  [Vd_Neg] -> Product/1
  Product/1 -> Sum/2
  Cos/1 -> [Cos]
  Sin/1 -> [Sin]
  [Vd_Pos] -> Sum/1
  Demux1/2 -> [Vq_Neg]
  Demux1/1 -> [Vd_Neg]
  Demux2/2 -> [Vq_Pos]
  Demux2/1 -> [Vd_Pos]
  Vdq_Inverse/1 -> Selector1/1
  Selector1/1 -> Demux1/1
  Selector/1 -> Demux2/1
  Vdq_in/1 -> Selector/1
  Gain/1 -> Sin/1, Cos/1
  Theta/1 -> Gain/1

== system GCI_Ctrl_PLL_C2000/C2000_SW/CtrlLoop/CurrentController/CurrentControllerPosNegSeq/Subsystem/abc_dqz/Subsystem ==
  abc : Inport  PortDimensions=3
  Gain1 : Gain  Gain=single(2/3)  ParamDataTypeStr=single  SaturateOnIntegerOverflow=on  OutDataTypeStr=Inherit: Same as input
  Gain3 : Gain  Gain="single([ 1   -1/2   -1/2; 0   sqrt(3)/2   -sqrt(3)/2; 1/2  1/2  1/2 ] )"  Multiplication=Matrix(K*u) (u vector)  ParamDataTypeStr=single  SaturateOnIntegerOverflow=on  OutDataTypeStr=Inherit: Same as input
  al_be_0 : Outport  VectorParamsAs1DForOutWhenUnconnected=off
  wires:
  abc/1 -> Gain3/1
  Gain3/1 -> Gain1/1
  Gain1/1 -> al_be_0/1

== system GCI_Ctrl_PLL_C2000/C2000_SW/CtrlLoop/CurrentController/CurrentControllerPosNegSeq/Subsystem/abc_dqz/Subsystem2 ==
  note: [  al
      |     be  ]
  note: q = -al*sin(wt) + be*cos(wt)
  note: [  cos(wt)   sin(wt)
      |    -sin(wt)    cos(wt)   ]
  note: d = al*cos(wt) + be*sin(wt)
  note: [ d
      |    q ]
  note: *
  note: =
  alpha_beta : Inport
  Ang : Inport  Port=2  PortDimensions=1
  Fcn : Fcn  Expr=u[1]*cos(u[3]) + u[2]*sin(u[3])
  Fcn1 : Fcn  Expr=-u[1]*sin(u[3]) + u[2]*cos(u[3])
  Mux : Mux  Inputs=3
  Mux1 : Mux  Inputs=[2 1]
  Mux2 : Mux  Inputs=[2 1]
  Selector : Selector  InputPortWidth=3  IndexOptions=Index vector (dialog)  Indices=[1 2]  OutputSizes=1
  Selector1 : Selector  InputPortWidth=3  IndexOptions=Index vector (dialog)  Indices=[3]  OutputSizes=1
  dq : Outport  InitialOutput=[0,0]  VectorParamsAs1DForOutWhenUnconnected=off
  wires:
  Selector1/1 -> Mux/3
  Selector/1 -> Mux1/1, Mux2/1
  Mux2/1 -> Fcn1/1
  Mux/1 -> dq/1
  Ang/1 -> Mux1/2, Mux2/2
  Fcn/1 -> Mux/1
  Fcn1/1 -> Mux/2
  Mux1/1 -> Fcn/1
  alpha_beta/1 -> Selector1/1, Selector/1

== system GCI_Ctrl_PLL_C2000/C2000_SW/CtrlLoop/CurrentController/CurrentControllerPosNegSeq/Subsystem/dd_dqz1/LPF ==
  u : Inport
  Alpha : Gain  Gain=(2-w*Ts)/(2+w*Ts)
  Beta : Gain  Gain=(w*Ts)/(2+w*Ts)
  Delay1 : Delay  DelayLength=1  InitialCondition=y_0
  Delay2 : Delay  DelayLength=1
  Sum1 : Sum  Inputs=++|
  Sum2 : Sum  Inputs=|++
  y : Outport  VectorParamsAs1DForOutWhenUnconnected=off
  wires:
  u/1 -> Sum1/1, Delay2/1
  Delay1/1 -> Alpha/1  "y(n-1)"
  Alpha/1 -> Sum2/2
  Delay2/1 -> Sum1/2
  Sum1/1 -> Beta/1
  Beta/1 -> Sum2/1
  Sum2/1 -> Delay1/1, y/1

== system GCI_Ctrl_PLL_C2000/C2000_SW/CtrlLoop/CurrentController/CurrentControllerPosNegSeq/Subsystem/dd_dqz1/LPF1 ==
  u : Inport
  Alpha : Gain  Gain=(2-w*Ts)/(2+w*Ts)
  Beta : Gain  Gain=(w*Ts)/(2+w*Ts)
  Delay1 : Delay  DelayLength=1  InitialCondition=y_0
  Delay2 : Delay  DelayLength=1
  Sum1 : Sum  Inputs=++|
  Sum2 : Sum  Inputs=|++
  y : Outport  VectorParamsAs1DForOutWhenUnconnected=off
  wires:
  Sum2/1 -> y/1, Delay1/1
  Beta/1 -> Sum2/1
  Sum1/1 -> Beta/1
  Delay2/1 -> Sum1/2
  Alpha/1 -> Sum2/2
  Delay1/1 -> Alpha/1  "y(n-1)"
  u/1 -> Delay2/1, Sum1/1

== system GCI_Ctrl_PLL_C2000/C2000_SW/CtrlLoop/CurrentController/CurrentControllerPosNegSeq/Subsystem/dd_dqz1/Subsystem ==
  abc : Inport  PortDimensions=3
  Gain1 : Gain  Gain=single(2/3)  ParamDataTypeStr=single  SaturateOnIntegerOverflow=on  OutDataTypeStr=Inherit: Same as input
  Gain3 : Gain  Gain="single([ 1   -1/2   -1/2; 0   sqrt(3)/2   -sqrt(3)/2; 1/2  1/2  1/2 ] )"  Multiplication=Matrix(K*u) (u vector)  ParamDataTypeStr=single  SaturateOnIntegerOverflow=on  OutDataTypeStr=Inherit: Same as input
  al_be_0 : Outport  VectorParamsAs1DForOutWhenUnconnected=off
  wires:
  abc/1 -> Gain3/1
  Gain3/1 -> Gain1/1
  Gain1/1 -> al_be_0/1  "AlphaBetaZero"

== system GCI_Ctrl_PLL_C2000/C2000_SW/CtrlLoop/CurrentController/CurrentControllerPosNegSeq/Subsystem/dd_dqz1/Subsystem1 ==
  note: =
  note: *
  note: [ d
      |    q ]
  note: d = al*cos(wt) + be*sin(wt)
  note: [  cos(wt)   sin(wt)
      |    -sin(wt)    cos(wt)   ]
  note: q = -al*sin(wt) + be*cos(wt)
  note: [  al
      |     be  ]
  alpha_beta : Inport
  wtNow : Inport  Port=2  PortDimensions=1
  Fcn : Fcn  Expr=u[1]*cos(u[3]) + u[2]*sin(u[3])
  Fcn1 : Fcn  Expr=-u[1]*sin(u[3]) + u[2]*cos(u[3])
  Mux : Mux  Inputs=3
  Mux1 : Mux  Inputs=[2 1]
  Mux2 : Mux  Inputs=[2 1]
  Selector : Selector  InputPortWidth=3  IndexOptions=Index vector (dialog)  Indices=[1 2]  OutputSizes=1
  Selector1 : Selector  InputPortWidth=3  IndexOptions=Index vector (dialog)  Indices=[3]  OutputSizes=1
  dq : Outport  InitialOutput=[0,0]  VectorParamsAs1DForOutWhenUnconnected=off
  wires:
  alpha_beta/1 -> Selector/1, Selector1/1
  Mux1/1 -> Fcn/1
  Fcn1/1 -> Mux/2
  Fcn/1 -> Mux/1
  wtNow/1 -> Mux2/2, Mux1/2
  Mux/1 -> dq/1
  Mux2/1 -> Fcn1/1
  Selector/1 -> Mux2/1, Mux1/1
  Selector1/1 -> Mux/3

== system GCI_Ctrl_PLL_C2000/C2000_SW/CtrlLoop/CurrentController/CurrentControllerPosNegSeq/Subsystem/dd_dqz1/Subsystem2 ==
  note: [  al
      |     be  ]
  note: q = -al*sin(wt) + be*cos(wt)
  note: [  cos(wt)   sin(wt)
      |    -sin(wt)    cos(wt)   ]
  note: d = al*cos(wt) + be*sin(wt)
  note: [ d
      |    q ]
  note: *
  note: =
  alpha_beta : Inport
  wtNow : Inport  Port=2  PortDimensions=1
  Fcn : Fcn  Expr=u[1]*cos(u[3]) + u[2]*sin(u[3])
  Fcn1 : Fcn  Expr=-u[1]*sin(u[3]) + u[2]*cos(u[3])
  Mux : Mux  Inputs=3
  Mux1 : Mux  Inputs=[2 1]
  Mux2 : Mux  Inputs=[2 1]
  Selector : Selector  InputPortWidth=3  IndexOptions=Index vector (dialog)  Indices=[1 2]  OutputSizes=1
  Selector1 : Selector  InputPortWidth=3  IndexOptions=Index vector (dialog)  Indices=[3]  OutputSizes=1
  dq : Outport  InitialOutput=[0,0]  VectorParamsAs1DForOutWhenUnconnected=off
  wires:
  Selector1/1 -> Mux/3
  Selector/1 -> Mux1/1, Mux2/1
  Mux2/1 -> Fcn1/1
  Mux/1 -> dq/1
  Fcn/1 -> Mux/1
  Fcn1/1 -> Mux/2
  Mux1/1 -> Fcn/1
  alpha_beta/1 -> Selector1/1, Selector/1
  wtNow/1 -> Mux2/2, Mux1/2

== system GCI_Ctrl_PLL_C2000/C2000_SW/CtrlLoop/CurrentController/CurrentControllerPosNegSeq/Subsystem/dd_dqz1/Subsystem3 ==
  Vdq_in : Inport
  Vdq_Inverse : Inport  Port=2
  Theta : Inport  Port=3
  Cos : Trigonometry  Operator=cos
  Cos1 : Trigonometry
  Demux1 : Demux  Outputs=2
  Demux2 : Demux  Outputs=2
  Gain : Gain  Gain=2  ParamDataTypeStr=single
  Ground : Ground
  Mux : Mux  Inputs=3
  Product{,1..3} (4 alike) : Product
  Selector : Selector  InputPortWidth=3  IndexOptions=Index vector (dialog)  Indices=[1 2]  OutputSizes=1
  Selector1 : Selector  InputPortWidth=3  IndexOptions=Index vector (dialog)  Indices=[1 2]  OutputSizes=1
  Sum : Sum  Inputs=|+-
  Sum1 : Sum  Inputs=|++
  Sum2 : Sum  Inputs=|+-
  Sum3 : Sum  Inputs=|+-
  Vdq_out : Outport  VectorParamsAs1DForOutWhenUnconnected=off
  wires:
  Ground/1 -> Mux/3
  Mux/1 -> Vdq_out/1
  Sum3/1 -> Mux/2
  Product3/1 -> Sum3/2
  Sum1/1 -> Sum3/1
  [Vq_Neg] -> Product3/1
  [Cos] -> Product3/2
  Product2/1 -> Sum2/2
  [Vq_Neg] -> Product2/1
  [Sin] -> Product2/2
  Sum2/1 -> Mux/1
  Sum/1 -> Sum2/1
  [Vq_Pos] -> Sum1/1
  Product1/1 -> Sum1/2
  [Vd_Neg] -> Product1/1
  [Sin] -> Product1/2
  [Cos] -> Product/2
  [Vd_Neg] -> Product/1
  Product/1 -> Sum/2
  Cos/1 -> [Cos]
  Cos1/1 -> [Sin]
  [Vd_Pos] -> Sum/1
  Demux1/2 -> [Vq_Neg]
  Demux1/1 -> [Vd_Neg]
  Demux2/2 -> [Vq_Pos]
  Demux2/1 -> [Vd_Pos]
  Vdq_Inverse/1 -> Selector1/1
  Selector1/1 -> Demux1/1
  Selector/1 -> Demux2/1
  Vdq_in/1 -> Selector/1
  Gain/1 -> Cos1/1, Cos/1
  Theta/1 -> Gain/1

== system GCI_Ctrl_PLL_C2000/C2000_SW/CtrlLoop/CurrentController/CurrentControllerPosNegSeq/Subsystem/dd_dqz1/Subsystem4 ==
  Vdq_in : Inport
  Vdq_Inverse : Inport  Port=2
  Theta : Inport  Port=3
  Cos : Trigonometry  Operator=cos
  Cos1 : Trigonometry
  Demux1 : Demux  Outputs=2
  Demux2 : Demux  Outputs=2
  Gain : Gain  Gain=2  ParamDataTypeStr=single
  Ground : Ground
  Mux : Mux  Inputs=3
  Product{,1..3} (4 alike) : Product
  Selector : Selector  InputPortWidth=3  IndexOptions=Index vector (dialog)  Indices=[1 2]  OutputSizes=1
  Selector1 : Selector  InputPortWidth=3  IndexOptions=Index vector (dialog)  Indices=[1 2]  OutputSizes=1
  Sum : Sum  Inputs=|+-
  Sum1 : Sum  Inputs=|++
  Sum2 : Sum  Inputs=|+-
  Sum3 : Sum  Inputs=|+-
  Vdq_out : Outport  VectorParamsAs1DForOutWhenUnconnected=off
  wires:
  Theta/1 -> Gain/1
  Gain/1 -> Cos1/1, Cos/1
  Vdq_in/1 -> Selector/1
  Selector/1 -> Demux2/1
  Selector1/1 -> Demux1/1
  Vdq_Inverse/1 -> Selector1/1
  Demux2/1 -> [Vd_Pos]
  Demux2/2 -> [Vq_Pos]
  Demux1/1 -> [Vd_Neg]
  Demux1/2 -> [Vq_Neg]
  [Vd_Pos] -> Sum/1
  Cos1/1 -> [Sin]
  Cos/1 -> [Cos]
  Product/1 -> Sum/2
  [Vd_Neg] -> Product/1
  [Cos] -> Product/2
  [Sin] -> Product1/2
  [Vd_Neg] -> Product1/1
  Product1/1 -> Sum1/2
  [Vq_Pos] -> Sum1/1
  Sum/1 -> Sum2/1
  Sum2/1 -> Mux/1
  [Sin] -> Product2/2
  [Vq_Neg] -> Product2/1
  Product2/1 -> Sum2/2
  [Cos] -> Product3/2
  [Vq_Neg] -> Product3/1
  Sum1/1 -> Sum3/1
  Product3/1 -> Sum3/2
  Sum3/1 -> Mux/2
  Mux/1 -> Vdq_out/1
  Ground/1 -> Mux/3

== system GCI_Ctrl_PLL_C2000/C2000_SW/CtrlLoop/CurrentController/CurrentControllerPosNegSeq/Subsystem/dd_dqz2/LPF ==
  u : Inport
  Alpha : Gain  Gain=(2-w*Ts)/(2+w*Ts)
  Beta : Gain  Gain=(w*Ts)/(2+w*Ts)
  Delay1 : Delay  DelayLength=1  InitialCondition=y_0
  Delay2 : Delay  DelayLength=1
  Sum1 : Sum  Inputs=++|
  Sum2 : Sum  Inputs=|++
  y : Outport  VectorParamsAs1DForOutWhenUnconnected=off
  wires:
  u/1 -> Sum1/1, Delay2/1
  Delay1/1 -> Alpha/1  "y(n-1)"
  Alpha/1 -> Sum2/2
  Delay2/1 -> Sum1/2
  Sum1/1 -> Beta/1
  Beta/1 -> Sum2/1
  Sum2/1 -> Delay1/1, y/1

== system GCI_Ctrl_PLL_C2000/C2000_SW/CtrlLoop/CurrentController/CurrentControllerPosNegSeq/Subsystem/dd_dqz2/LPF1 ==
  u : Inport
  Alpha : Gain  Gain=(2-w*Ts)/(2+w*Ts)
  Beta : Gain  Gain=(w*Ts)/(2+w*Ts)
  Delay1 : Delay  DelayLength=1  InitialCondition=y_0
  Delay2 : Delay  DelayLength=1
  Sum1 : Sum  Inputs=++|
  Sum2 : Sum  Inputs=|++
  y : Outport  VectorParamsAs1DForOutWhenUnconnected=off
  wires:
  Sum2/1 -> y/1, Delay1/1
  Beta/1 -> Sum2/1
  Sum1/1 -> Beta/1
  Delay2/1 -> Sum1/2
  Alpha/1 -> Sum2/2
  Delay1/1 -> Alpha/1  "y(n-1)"
  u/1 -> Delay2/1, Sum1/1

== system GCI_Ctrl_PLL_C2000/C2000_SW/CtrlLoop/CurrentController/CurrentControllerPosNegSeq/Subsystem/dd_dqz2/Subsystem ==
  abc : Inport  PortDimensions=3
  Gain1 : Gain  Gain=single(2/3)  ParamDataTypeStr=single  SaturateOnIntegerOverflow=on  OutDataTypeStr=Inherit: Same as input
  Gain3 : Gain  Gain="single([ 1   -1/2   -1/2; 0   sqrt(3)/2   -sqrt(3)/2; 1/2  1/2  1/2 ] )"  Multiplication=Matrix(K*u) (u vector)  ParamDataTypeStr=single  SaturateOnIntegerOverflow=on  OutDataTypeStr=Inherit: Same as input
  al_be_0 : Outport  VectorParamsAs1DForOutWhenUnconnected=off
  wires:
  Gain1/1 -> al_be_0/1  "AlphaBetaZero"
  Gain3/1 -> Gain1/1
  abc/1 -> Gain3/1

== system GCI_Ctrl_PLL_C2000/C2000_SW/CtrlLoop/CurrentController/CurrentControllerPosNegSeq/Subsystem/dd_dqz2/Subsystem1 ==
  note: [  al
      |     be  ]
  note: q = -al*sin(wt) + be*cos(wt)
  note: [  cos(wt)   sin(wt)
      |    -sin(wt)    cos(wt)   ]
  note: d = al*cos(wt) + be*sin(wt)
  note: [ d
      |    q ]
  note: *
  note: =
  alpha_beta : Inport
  wtNow : Inport  Port=2  PortDimensions=1
  Fcn : Fcn  Expr=u[1]*cos(u[3]) + u[2]*sin(u[3])
  Fcn1 : Fcn  Expr=-u[1]*sin(u[3]) + u[2]*cos(u[3])
  Mux : Mux  Inputs=3
  Mux1 : Mux  Inputs=[2 1]
  Mux2 : Mux  Inputs=[2 1]
  Selector : Selector  InputPortWidth=3  IndexOptions=Index vector (dialog)  Indices=[1 2]  OutputSizes=1
  Selector1 : Selector  InputPortWidth=3  IndexOptions=Index vector (dialog)  Indices=[3]  OutputSizes=1
  dq : Outport  InitialOutput=[0,0]  VectorParamsAs1DForOutWhenUnconnected=off
  wires:
  Selector1/1 -> Mux/3
  Selector/1 -> Mux1/1, Mux2/1
  Mux2/1 -> Fcn1/1
  Mux/1 -> dq/1  "dq"
  wtNow/1 -> Mux1/2, Mux2/2
  Fcn/1 -> Mux/1
  Fcn1/1 -> Mux/2
  Mux1/1 -> Fcn/1
  alpha_beta/1 -> Selector1/1, Selector/1

== system GCI_Ctrl_PLL_C2000/C2000_SW/CtrlLoop/CurrentController/CurrentControllerPosNegSeq/Subsystem/dd_dqz2/Subsystem2 ==
  note: =
  note: *
  note: [ d
      |    q ]
  note: d = al*cos(wt) + be*sin(wt)
  note: [  cos(wt)   sin(wt)
      |    -sin(wt)    cos(wt)   ]
  note: q = -al*sin(wt) + be*cos(wt)
  note: [  al
      |     be  ]
  alpha_beta : Inport
  wtNow : Inport  Port=2  PortDimensions=1
  Fcn : Fcn  Expr=u[1]*cos(u[3]) + u[2]*sin(u[3])
  Fcn1 : Fcn  Expr=-u[1]*sin(u[3]) + u[2]*cos(u[3])
  Mux : Mux  Inputs=3
  Mux1 : Mux  Inputs=[2 1]
  Mux2 : Mux  Inputs=[2 1]
  Selector : Selector  InputPortWidth=3  IndexOptions=Index vector (dialog)  Indices=[1 2]  OutputSizes=1
  Selector1 : Selector  InputPortWidth=3  IndexOptions=Index vector (dialog)  Indices=[3]  OutputSizes=1
  dq : Outport  InitialOutput=[0,0]  VectorParamsAs1DForOutWhenUnconnected=off
  wires:
  alpha_beta/1 -> Selector/1, Selector1/1
  Mux1/1 -> Fcn/1
  Fcn1/1 -> Mux/2
  Fcn/1 -> Mux/1
  wtNow/1 -> Mux2/2, Mux1/2
  Mux/1 -> dq/1  "dq"
  Mux2/1 -> Fcn1/1
  Selector/1 -> Mux2/1, Mux1/1
  Selector1/1 -> Mux/3

== system GCI_Ctrl_PLL_C2000/C2000_SW/CtrlLoop/CurrentController/CurrentControllerPosNegSeq/Subsystem/dd_dqz2/Subsystem3 ==
  Vdq_in : Inport
  Vdq_Inverse : Inport  Port=2
  Theta : Inport  Port=3
  Cos : Trigonometry  Operator=cos
  Demux1 : Demux  Outputs=2
  Demux2 : Demux  Outputs=2
  Gain : Gain  Gain=2  ParamDataTypeStr=single
  Ground : Ground
  Mux : Mux  Inputs=3
  Product{,1..3} (4 alike) : Product
  Selector : Selector  InputPortWidth=3  IndexOptions=Index vector (dialog)  Indices=[1 2]  OutputSizes=1
  Selector1 : Selector  InputPortWidth=3  IndexOptions=Index vector (dialog)  Indices=[1 2]  OutputSizes=1
  Sin : Trigonometry
  Sum : Sum  Inputs=|+-
  Sum1 : Sum  Inputs=|++
  Sum2 : Sum  Inputs=|+-
  Sum3 : Sum  Inputs=|+-
  Vdq_out : Outport  VectorParamsAs1DForOutWhenUnconnected=off
  wires:
  Theta/1 -> Gain/1
  Gain/1 -> Cos/1, Sin/1
  Vdq_in/1 -> Selector/1
  Selector/1 -> Demux2/1
  Selector1/1 -> Demux1/1
  Vdq_Inverse/1 -> Selector1/1
  Demux2/1 -> [Vd_Pos]
  Demux2/2 -> [Vq_Pos]
  Demux1/1 -> [Vd_Neg]
  Demux1/2 -> [Vq_Neg]
  [Vd_Pos] -> Sum/1
  Sin/1 -> [Sin]
  Cos/1 -> [Cos]
  Product/1 -> Sum/2
  [Vd_Neg] -> Product/1
  [Cos] -> Product/2
  [Sin] -> Product1/2
  [Vd_Neg] -> Product1/1
  Product1/1 -> Sum1/2
  [Vq_Pos] -> Sum1/1
  Sum/1 -> Sum2/1
  Sum2/1 -> Mux/1
  [Sin] -> Product2/2
  [Vq_Neg] -> Product2/1
  Product2/1 -> Sum2/2
  [Cos] -> Product3/2
  [Vq_Neg] -> Product3/1
  Sum1/1 -> Sum3/1
  Product3/1 -> Sum3/2
  Sum3/1 -> Mux/2
  Mux/1 -> Vdq_out/1
  Ground/1 -> Mux/3

== system GCI_Ctrl_PLL_C2000/C2000_SW/CtrlLoop/CurrentController/CurrentControllerPosNegSeq/Subsystem/dd_dqz2/Subsystem4 ==
  Vdq_in : Inport
  Vdq_Inverse : Inport  Port=2
  Theta : Inport  Port=3
  Cos : Trigonometry  Operator=cos
  Demux1 : Demux  Outputs=2
  Demux2 : Demux  Outputs=2
  Gain : Gain  Gain=2  ParamDataTypeStr=single
  Ground : Ground
  Mux : Mux  Inputs=3
  Product{,1..3} (4 alike) : Product
  Selector : Selector  InputPortWidth=3  IndexOptions=Index vector (dialog)  Indices=[1 2]  OutputSizes=1
  Selector1 : Selector  InputPortWidth=3  IndexOptions=Index vector (dialog)  Indices=[1 2]  OutputSizes=1
  Sin : Trigonometry
  Sum : Sum  Inputs=|+-
  Sum1 : Sum  Inputs=|++
  Sum2 : Sum  Inputs=|+-
  Sum3 : Sum  Inputs=|+-
  Vdq_out : Outport  VectorParamsAs1DForOutWhenUnconnected=off
  wires:
  Ground/1 -> Mux/3
  Mux/1 -> Vdq_out/1
  Sum3/1 -> Mux/2
  Product3/1 -> Sum3/2
  Sum1/1 -> Sum3/1
  [Vq_Neg] -> Product3/1
  [Cos] -> Product3/2
  Product2/1 -> Sum2/2
  [Vq_Neg] -> Product2/1
  [Sin] -> Product2/2
  Sum2/1 -> Mux/1
  Sum/1 -> Sum2/1
  [Vq_Pos] -> Sum1/1
  Product1/1 -> Sum1/2
  [Vd_Neg] -> Product1/1
  [Sin] -> Product1/2
  [Cos] -> Product/2
  [Vd_Neg] -> Product/1
  Product/1 -> Sum/2
  Cos/1 -> [Cos]
  Sin/1 -> [Sin]
  [Vd_Pos] -> Sum/1
  Demux1/2 -> [Vq_Neg]
  Demux1/1 -> [Vd_Neg]
  Demux2/2 -> [Vq_Pos]
  Demux2/1 -> [Vd_Pos]
  Vdq_Inverse/1 -> Selector1/1
  Selector1/1 -> Demux1/1
  Selector/1 -> Demux2/1
  Vdq_in/1 -> Selector/1
  Gain/1 -> Sin/1, Cos/1
  Theta/1 -> Gain/1

== system GCI_Ctrl_PLL_C2000/C2000_SW/CtrlLoop/CurrentController/FeedForward/Subsystem/abc_dqz/Subsystem ==
  abc : Inport  PortDimensions=3
  Gain1 : Gain  Gain=single(2/3)  ParamDataTypeStr=single  SaturateOnIntegerOverflow=on  OutDataTypeStr=Inherit: Same as input
  Gain3 : Gain  Gain="single([ 1   -1/2   -1/2; 0   sqrt(3)/2   -sqrt(3)/2; 1/2  1/2  1/2 ] )"  Multiplication=Matrix(K*u) (u vector)  ParamDataTypeStr=single  SaturateOnIntegerOverflow=on  OutDataTypeStr=Inherit: Same as input
  al_be_0 : Outport  VectorParamsAs1DForOutWhenUnconnected=off
  wires:
  abc/1 -> Gain3/1
  Gain3/1 -> Gain1/1
  Gain1/1 -> al_be_0/1
